simulink model "MPC_test"  (R2020a)
settings: Solver=FixedStepAuto  StartTime=0.0  StopTime=100  FixedStep=0.01  MaxStep=0.01  RelTol=1e-3
InitFcn:
  | MPC_test_setup
values from neighbouring files (symbols this model uses):
  A = real(A)    [MPC_test_setup.m]    (also in generate_toy_model.m; online_DMD.m)
  A_hat = AB(:,1:q*ny)    [MPC_test_setup.m]    (also in generate_toy_model.m = AB(:,1:q*m))
  B = AB(:,(ny+1):end)    [online_DMD.m]
  B_hat = AB(:,(q*ny+1):end)    [MPC_test_setup.m]    (also in generate_toy_model.m = AB(:,(q*m+1):end))
  C_hat = eye(m_hat)    [MPC_test_setup.m]    (also in generate_toy_model.m)
  C_plant = eye(3)    [MPC_test_setup.m]    (also in generate_toy_model.m)
  D = (q-1)*Ts    [MPC_test_setup.m]    (also in generate_toy_model.m)
  D_hat = zeros(m_hat, l_hat)    [MPC_test_setup.m]    (also in generate_toy_model.m)
  D_plant = zeros(3,2)    [MPC_test_setup.m]    (also in generate_toy_model.m)
  Ts = t(2)-t(1)    [MPC_test_setup.m]    (also in generate_toy_model.m; online_DMD.m)
  U_nom = u_bar    [MPC_test_setup.m]    (also in generate_toy_model.m)
  x0 = zeros(3,1)    [MPC_test_setup.m]    (also in generate_toy_model.m)
  x0_hat = zeros(n_hat,1)    [MPC_test_setup.m]    (also in generate_toy_model.m)
  X_nom = zeros(n_hat,1)    [MPC_test_setup.m]    (also in generate_toy_model.m)
  Y = zeros(q*ny,w)    [MPC_test_setup.m]    (also in generate_toy_model.m = zeros(q*m,w); online_DMD.m = [Y(:,2:end), y])
  Y_nom = zeros(m_hat,1)    [MPC_test_setup.m]    (also in generate_toy_model.m)
undefined symbols (not defined in the file or in its folder): A_plant, B_plant, C, DX, DX_hat, U, X
libraries: mpclib x2
settings Model: Creator=murray  LastModifiedBy=murray

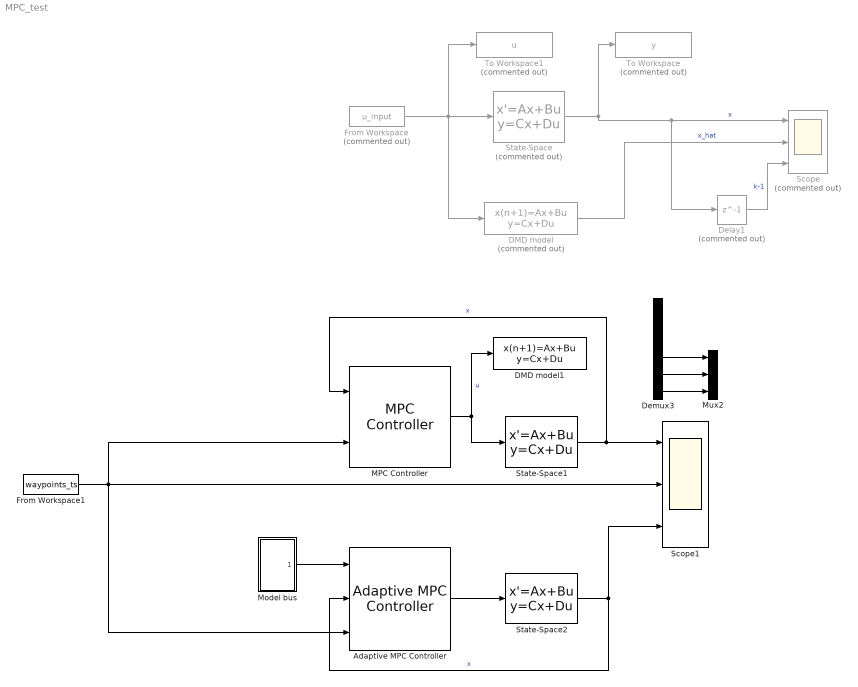
== system MPC_test ==
  Adaptive MPC Controller : mpclib/Adaptive MPC Controller  SCDEnableBlockLinearizationSpecification=on  mpcobj=MPCobj  enable_value=0  updateMPCinCallerWorkspace=on  md_inport=off  mv_inport=off  uref_inport=off  return_cost=off  return_mvseq=off  return_qpstatus=off  return_xseq=off  return_state=off  return_ovseq=off  state_inport=off  isltv_plant=off  umin_inport=off  umax_inport=off  ymin_inport=off  ymax_inport=off  cc_inport=off  ywt_inport=off  uwt_inport=off  duwt_inport=off  rhoeps_inport=off  pm_inport=off  MaximumP=10  HorizonChoice=FixedHorizon  BlockDataType=double  SampleTimeInherited=off  switch_inport=off
  DMD model : DiscreteStateSpace  Commented=on  A=A_hat  B=B_hat  C=C_hat  D=D_hat  InitialCondition=x0_hat  SampleTime=Ts
  DMD model1 : DiscreteStateSpace  A=A_hat  B=B_hat  C=C_hat  D=D_hat  InitialCondition=x0_hat  SampleTime=Ts
  Delay1 : Delay  Commented=on  DelayLength=1  SampleTime=Ts
  Demux3 : Demux  Outputs=6
  From Workspace : FromWorkspace  Commented=on  VariableName=u_input
  From Workspace1 : FromWorkspace  VariableName=waypoints_ts
  MPC Controller : mpclib/MPC Controller  SCDEnableBlockLinearizationSpecification=on  mpcobj=MPCobj  is_multiple=0  enable_value=0  return_u0=off  updateMPCinCallerWorkspace=on  md_inport=off  mv_inport=off  uref_inport=off  return_cost=off  return_mvseq=off  return_qpstatus=off  return_xseq=off  return_state=off  return_ovseq=off  state_inport=off  umin_inport=off  umax_inport=off  ymin_inport=off  ymax_inport=off  cc_inport=off  ywt_inport=off  uwt_inport=off  duwt_inport=off  rhoeps_inport=off  pm_inport=off  MaximumP=10  HorizonChoice=FixedHorizon  n_ts=0.1  n_p=10  n_mv=2  n_md=0  n_ud=0  n_mo=6  n_uo=0  BlockDataType=double  SampleTimeInherited=off  switch_inport=off
  Model bus : Subsystem
  Mux2 : Mux  Inputs=3
  Scope : Scope  Commented=on  NumInputPorts=3
  Scope1 : Scope  NumInputPorts=3
  State-Space : StateSpace  Commented=on  A=A_plant  B=B_plant  C=eye(3)  D=zeros(3,2)  InitialCondition=zeros(3,1)
  State-Space1 : StateSpace  A=A_plant  B=B_plant  C=C_plant  D=D_plant  InitialCondition=x0
  State-Space2 : StateSpace  A=A_plant  B=B_plant  C=C_plant  D=D_plant  InitialCondition=x0
  To Workspace : ToWorkspace  Commented=on  VariableName=y  SaveFormat=Timeseries  SampleTime=-1
  To Workspace1 : ToWorkspace  Commented=on  VariableName=u  SaveFormat=Timeseries  SampleTime=-1
  wires:
  From Workspace/1 -> DMD model/1, To Workspace1/1, State-Space/1
  State-Space/1 -> To Workspace/1, Delay1/1, Scope/1  "x"
  MPC Controller/1 -> DMD model1/1, State-Space1/1  "u"
  Delay1/1 -> Scope/3  "k-1"
  DMD model/1 -> Scope/2  "x_hat"
  From Workspace1/1 -> Adaptive MPC Controller/3, Scope1/2, MPC Controller/2
  Demux3/4 -> Mux2/1
  Demux3/5 -> Mux2/2
  Demux3/6 -> Mux2/3
  State-Space1/1 -> MPC Controller/1, Scope1/1  "x"
  Adaptive MPC Controller/1 -> State-Space2/1
  State-Space2/1 -> Scope1/3, Adaptive MPC Controller/2  "x"
  Model bus/1(model) -> Adaptive MPC Controller/1

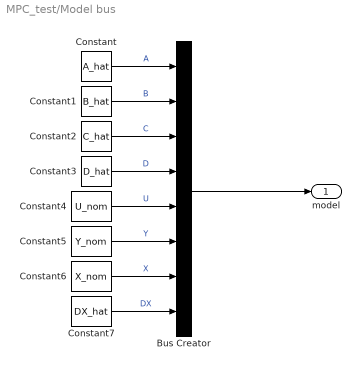
== system MPC_test/Model bus ==
  Bus Creator : BusCreator  Inputs=A,B,C,D,X,Y,U,DX
  Constant : Constant  Value=A_hat
  Constant1 : Constant  Value=B_hat
  Constant2 : Constant  Value=C_hat
  Constant3 : Constant  Value=D_hat
  Constant4 : Constant  Value=U_nom
  Constant5 : Constant  Value=Y_nom
  Constant6 : Constant  Value=X_nom
  Constant7 : Constant  Value=DX_hat
  model : Outport
  wires:
  Constant/1 -> Bus Creator/1  "A"
  Constant7/1 -> Bus Creator/8  "DX"
  Constant5/1 -> Bus Creator/6  "Y"
  Constant3/1 -> Bus Creator/4  "D"
  Constant1/1 -> Bus Creator/2  "B"
  Constant2/1 -> Bus Creator/3  "C"
  Bus Creator/1 -> model/1
  Constant6/1 -> Bus Creator/7  "X"
  Constant4/1 -> Bus Creator/5  "U"
